simulink model "EE17BTECH11001"  (R2018b)
settings: Solver=VariableStepAuto  StartTime=0.0  StopTime=10.0  RelTol=1e-3
libraries: powerlib x20, simulink x1
settings Model: Creator=ALLA BROTHERS  LastModifiedBy=ALLA BROTHERS

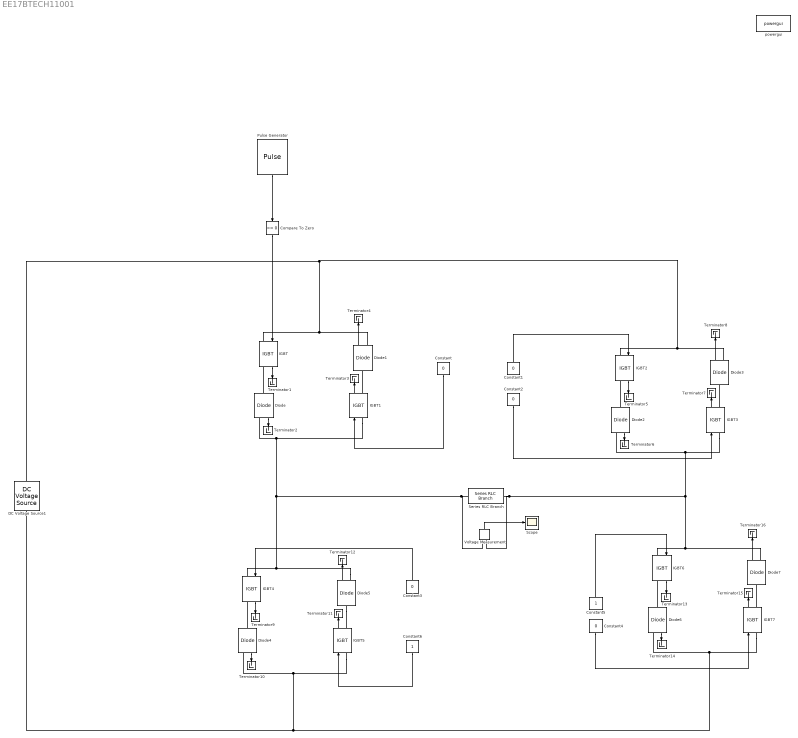
== system EE17BTECH11001 ==
  Compare To Zero : simulink/Logic and Bit Operations/Compare To Zero  relop=<=  OutDataTypeStr=boolean
  Constant{,1..4} (5 alike) : Constant  Value=0
  Constant5 : Constant
  Constant6 : Constant
  DC Voltage Source1 : powerlib/Electrical Sources/DC Voltage Source  Amplitude=30  Measurements=None
  Diode{,1..7} (8 alike) : powerlib/Power Electronics/Diode  Ron=0.001  Lon=0  Vf=0.8  IC=0  UseSnubber=0  Rs=500  Cs=250e-9  Measurements=on
  IGBT{,1..7} (8 alike) : powerlib/Power Electronics/IGBT  Ron=0.001  Lon=0  Vf=1  Tf=1e-6  Tt=2e-6  IC=0  Rs=1e5  Cs=inf  Measurements=on
  Pulse Generator : DiscretePulseGenerator  PulseType=Time based  Period=0.02  PulseWidth=50
  Scope : Scope
  Series RLC Branch : powerlib/Elements/Series RLC Branch  LConnTagsString=__new0  RConnTagsString=__new0  BranchType=RLC  Resistance=50  Inductance=4e-3  SetiL0=off  InitialCurrent=0  Capacitance=0  Setx0=off  InitialVoltage=0  Measurements=None
  Terminator{1..16} (16 alike) : Terminator
  Voltage Measurement : powerlib/Measurements/Voltage Measurement  PhasorSimulation=off  OutputType=Complex  PSBequivalent=0
  powergui : powerlib/powergui  Priority=1  SimulationMode=Continuous  SampleTime=50e-6  frequency=60  Iterations=50  frequencyindice=0  Pbase=100e6  ErrMax=1e-4  UnitsV=kV  UnitsW=MW  buscounter=0  FunctionMessages=off  echomessages=off  EnableUseOfTLC=off  CurrentSourceSwitches=off  DisableSnubberDevices=off  DisableRonSwitches=off  DisableVfSwitches=off  DisplayEquations=off  SolverType=Tustin/Backward Euler (TBE)  Interpol=off  ExternalGateDelay=off  methode=off  Ts=100  x0status=blocks  SPID=on  SwTol=0  HookPort=off  RestoreLinks=warning  ResistiveCurrentMeasurement=off  Frange=[0:2:500]  Ylog=off  Xlog=on  ShowGrid=off  save=off  variable=ZData  structure=0  ZoomFFT=off  StartTime=0.0  cycles=1  DisplayStyle=1  fundamental=60  FreqAxis=off  MaxFrequency=1000  frequencyindicesteady=1  RmsSteady=1  display=off
  wires:
  Diode/1 -> Terminator2/1
  IGBT1/1 -> Terminator3/1
  Diode1/1 -> Terminator4/1
  IGBT/1 -> Terminator1/1
  Constant/1 -> IGBT1/1
  IGBT3/1 -> Terminator7/1
  Constant1/1 -> IGBT2/1
  Diode2/1 -> Terminator6/1
  Constant2/1 -> IGBT3/1
  Diode3/1 -> Terminator8/1
  IGBT2/1 -> Terminator5/1
  Constant4/1 -> IGBT7/1
  Constant5/1 -> IGBT6/1
  Diode7/1 -> Terminator16/1
  Diode6/1 -> Terminator14/1
  IGBT6/1 -> Terminator13/1
  IGBT7/1 -> Terminator15/1
  Diode5/1 -> Terminator12/1
  Constant6/1 -> IGBT5/1
  IGBT4/1 -> Terminator9/1
  IGBT5/1 -> Terminator11/1
  Constant3/1 -> IGBT4/1
  Diode4/1 -> Terminator10/1
  Voltage Measurement/1 -> Scope/1
  Compare To Zero/1 -> IGBT/1
  Pulse Generator/1 -> Compare To Zero/1
  connections:
  IGBT1/RConn1 -- Diode1/LConn1
  Diode5/RConn1 -- IGBT4/LConn1 -- Voltage Measurement/LConn1 -- Series RLC Branch/LConn1 -- IGBT1/LConn1 -- Diode/RConn1
  Diode/LConn1 -- IGBT/RConn1
  IGBT3/RConn1 -- Diode3/LConn1
  Diode2/LConn1 -- IGBT2/RConn1
  IGBT/LConn1 -- Diode1/RConn1 -- DC Voltage Source1/RConn1 -- Diode3/RConn1 -- IGBT2/LConn1
  IGBT3/LConn1 -- Diode2/RConn1 -- Voltage Measurement/LConn2 -- Series RLC Branch/RConn1 -- Diode7/RConn1 -- IGBT6/LConn1
  IGBT5/LConn1 -- DC Voltage Source1/LConn1 -- Diode6/RConn1 -- IGBT7/LConn1 -- Diode4/RConn1
  Diode6/LConn1 -- IGBT6/RConn1
  IGBT7/RConn1 -- Diode7/LConn1
  Diode4/LConn1 -- IGBT4/RConn1
  Diode5/LConn1 -- IGBT5/RConn1
